simulink model "pcssp_KCURR_PFPO1_for_MUSCLE3"  (R2023b)
settings: configuration reference "configurationSettings" (kept outside this file)
undefined symbols (not defined in the file or in its folder): DiscIntNeverNeededParam, KCURR_PFPO1_fp, KCURR_PFPO1_tp, ParameterScheduling_KCURR, PCSSP_KCURR_ext_sizes
libraries: simulink x4
(part 1 of 2)
Description:
  | The KCURR_PFPO1 module implements a CS/PF current controller, including control of IpThis version performs internal gain scheduling based on an externally fed scheduling variable. Note: the coils are sorted as CS3U CS2U CS1 CS2L CS3L P1 P2 P3 P4 P5 P6
settings Model: DataDictionary=pcssp_KCURR_PFPO1.sldd  Creator=ravenst1  LastModifiedBy=grosg1
settings ConfigSetRef: SourceName=configurationSettings

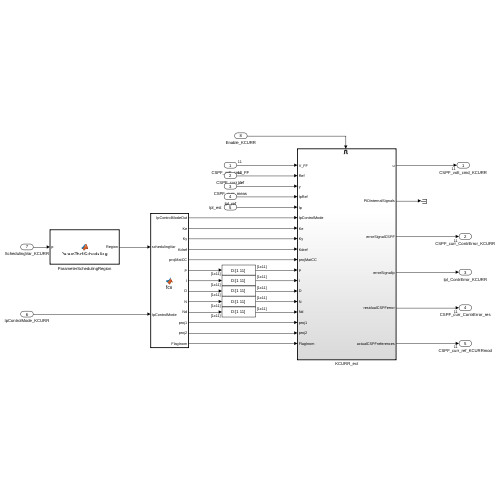
[thumbnail: Simulink's stored preview of the top-level diagram]
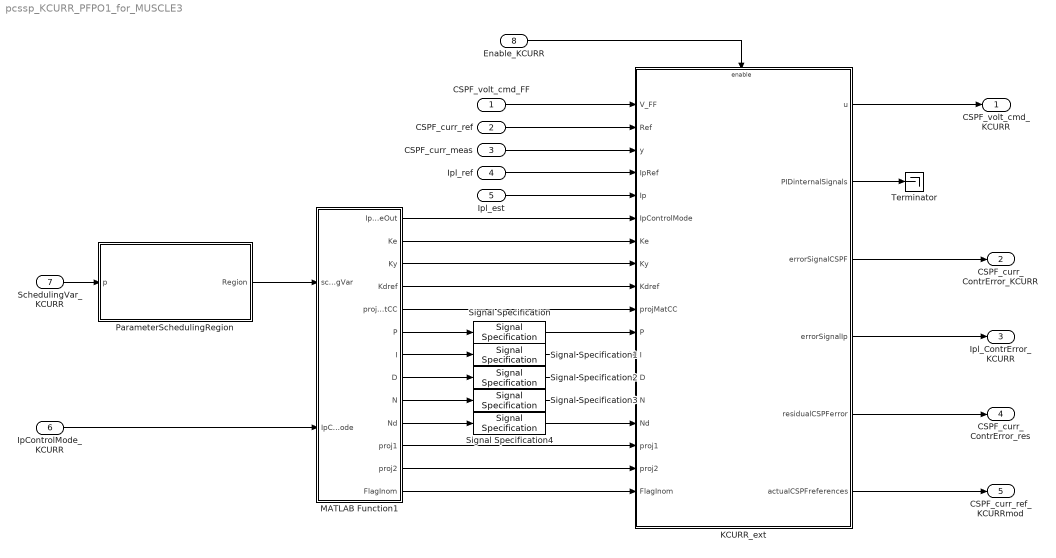
== system pcssp_KCURR_PFPO1_for_MUSCLE3 ==
  CSPF_volt_cmd_FF : Inport  PortDimensions=PCSSP_KCURR_ext_sizes.CSPF  SampleTime=KCURR_PFPO1_fp.Ts
  CSPF_curr_ref : Inport  Port=2  PortDimensions=PCSSP_KCURR_ext_sizes.CSPF  SampleTime=KCURR_PFPO1_fp.Ts
  CSPF_curr_meas : Inport  Port=3  PortDimensions=PCSSP_KCURR_ext_sizes.CSPF  SampleTime=KCURR_PFPO1_fp.Ts
  Ipl_ref : Inport  Port=4  SampleTime=KCURR_PFPO1_fp.Ts
  Ipl_est : Inport  Port=5  SampleTime=KCURR_PFPO1_fp.Ts
  IpControlMode_KCURR : Inport  Port=6  SampleTime=KCURR_PFPO1_fp.Ts
  SchedulingVar_KCURR : Inport  Port=7  PortDimensions=PCSSP_KCURR_ext_sizes.scheduling_var  SampleTime=KCURR_PFPO1_fp.Ts
  Enable_KCURR : Inport  Port=8
  KCURR_ext : Subsystem
  MATLAB Function1 : MATLAB Function  TreatAsAtomicUnit=on
  ParameterSchedulingRegion : MATLAB Function  TreatAsAtomicUnit=on
  Signal Specification{,1..4} (5 alike) : SignalSpecification  Dimensions=[1 11]
  Terminator : Terminator
  CSPF_volt_cmd_KCURR : Outport  PortDimensions=PCSSP_KCURR_ext_sizes.CSPF
  CSPF_curr_ContrError_KCURR : Outport  Port=2  PortDimensions=PCSSP_KCURR_ext_sizes.CSPF
  Ipl_ContrError_KCURR : Outport  Port=3  PortDimensions=1
  CSPF_curr_ContrError_res : Outport  Port=4  PortDimensions=PCSSP_KCURR_ext_sizes.CSPF
  CSPF_curr_ref_KCURRmod : Outport  Port=5  PortDimensions=PCSSP_KCURR_ext_sizes.CSPF
  wires:
  MATLAB Function1/10(Nd) -> Signal Specification4/1
  CSPF_curr_meas/1 -> KCURR_ext/3(y)
  MATLAB Function1/13(FlagInom) -> KCURR_ext/18(FlagInom)
  MATLAB Function1/12(proj2) -> KCURR_ext/17(proj2)
  Enable_KCURR/1 -> KCURR_ext/Enable
  MATLAB Function1/5(projMatCC) -> KCURR_ext/10(projMatCC)
  MATLAB Function1/1(IpControlModeOut) -> KCURR_ext/6(IpControlMode)
  Ipl_est/1 -> KCURR_ext/5(Ip)
  CSPF_curr_ref/1 -> KCURR_ext/2(Ref)
  ParameterSchedulingRegion/1(Region) -> MATLAB Function1/1(schedulingVar)
  CSPF_volt_cmd_FF/1 -> KCURR_ext/1(V_FF)
  MATLAB Function1/3(Ky) -> KCURR_ext/8(Ky)
  MATLAB Function1/9(N) -> Signal Specification3/1
  MATLAB Function1/4(Kdref) -> KCURR_ext/9(Kdref)
  SchedulingVar_KCURR/1 -> ParameterSchedulingRegion/1(p)
  MATLAB Function1/2(Ke) -> KCURR_ext/7(Ke)
  Ipl_ref/1 -> KCURR_ext/4(IpRef)
  IpControlMode_KCURR/1 -> MATLAB Function1/2(IpControlMode)
  MATLAB Function1/6(P) -> Signal Specification/1
  Signal Specification/1 -> KCURR_ext/11(P)
  Signal Specification1/1 -> KCURR_ext/12(I)
  MATLAB Function1/7(I) -> Signal Specification1/1
  Signal Specification2/1 -> KCURR_ext/13(D)
  MATLAB Function1/8(D) -> Signal Specification2/1
  Signal Specification3/1 -> KCURR_ext/14(N)
  Signal Specification4/1 -> KCURR_ext/15(Nd)
  MATLAB Function1/11(proj1) -> KCURR_ext/16(proj1)
  KCURR_ext/1(u) -> CSPF_volt_cmd_KCURR/1
  KCURR_ext/2(PIDinternalSignals) -> Terminator/1
  KCURR_ext/3(errorSignalCSPF) -> CSPF_curr_ContrError_KCURR/1
  KCURR_ext/4(errorSignalIp) -> Ipl_ContrError_KCURR/1
  KCURR_ext/5(residualCSPFerror) -> CSPF_curr_ContrError_res/1
  KCURR_ext/6(actualCSPFreferences) -> CSPF_curr_ref_KCURRmod/1

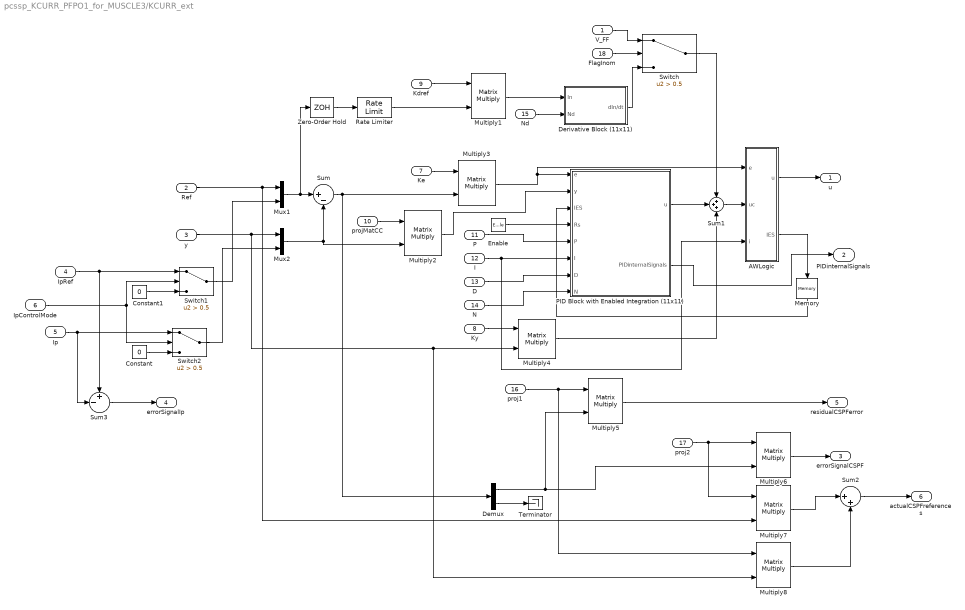
== system pcssp_KCURR_PFPO1_for_MUSCLE3/KCURR_ext ==
  V_FF : Inport
  Ref : Inport  Port=2
  y : Inport  Port=3
  IpRef : Inport  Port=4
  Ip : Inport  Port=5
  IpControlMode : Inport  Port=6
  Ke : Inport  Port=7
  Ky : Inport  Port=8
  Kdref : Inport  Port=9
  projMatCC : Inport  Port=10
  P : Inport  Port=11
  I : Inport  Port=12
  D : Inport  Port=13
  N : Inport  Port=14
  Nd : Inport  Port=15
  proj1 : Inport  Port=16
  proj2 : Inport  Port=17
  FlagInom : Inport  Port=18
  Enable : EnablePort  StatesWhenEnabling=reset  ShowOutputPort=on
  AWLogic : Subsystem
  Constant : Constant  Value=0
  Constant1 : Constant  Value=0
  Demux : Demux  Outputs=[11 1]
  Derivative Block (11x11) : Subsystem
  Memory : Memory
  Multiply{1..8} (8 alike) : Product  Inputs=**  Multiplication=Matrix(*)
  Mux1 : Mux  Inputs=2
  Mux2 : Mux  Inputs=2
  "PID Block with Enabled Integration (11x11) " : Subsystem
  Rate Limiter : RateLimiter  RisingSlewLimit=KCURR_PFPO1_tp.PosCurSlewRate  FallingSlewLimit=KCURR_PFPO1_tp.NegCurSlewRate  SampleTimeMode=inherited
  Sum : Sum  Inputs=|+-
  Sum1 : Sum  Inputs=+++
  Sum2 : Sum  Inputs=|++
  Sum3 : Sum  Inputs=+-|
  Switch : Switch  Criteria=u2 > Threshold  Threshold=0.5  SaturateOnIntegerOverflow=off  InputSameDT=off
  Switch1 : Switch  Criteria=u2 > Threshold  Threshold=0.5  SaturateOnIntegerOverflow=off  InputSameDT=off
  Switch2 : Switch  Criteria=u2 > Threshold  Threshold=0.5  SaturateOnIntegerOverflow=off  InputSameDT=off
  Terminator : Terminator
  Zero-Order Hold : ZeroOrderHold  SampleTime=KCURR_PFPO1_fp.Ts
  u : Outport
  PIDinternalSignals : Outport  Port=2
  errorSignalCSPF : Outport  Port=3
  errorSignalIp : Outport  Port=4
  residualCSPFerror : Outport  Port=5
  actualCSPFreferences : Outport  Port=6
  wires:
  N/1 -> "PID Block with Enabled Integration (11x11) "/8(N)
  D/1 -> "PID Block with Enabled Integration (11x11) "/7(D)
  I/1 -> "PID Block with Enabled Integration (11x11) "/6(I), AWLogic/3(i)
  P/1 -> "PID Block with Enabled Integration (11x11) "/5(P)
  Nd/1 -> Derivative Block (11x11)/2(Nd)
  Multiply3/1 -> AWLogic/1(e), "PID Block with Enabled Integration (11x11) "/1(e)
  "PID Block with Enabled Integration (11x11) "/2(PIDinternalSignals) -> PIDinternalSignals/1
  "PID Block with Enabled Integration (11x11) "/1(u) -> Sum1/2
  Multiply4/1 -> Sum1/3
  V_FF/1 -> Switch/1
  Switch/1 -> Sum1/1
  FlagInom/1 -> Switch/2
  Kdref/1 -> Multiply1/1
  Ke/1 -> Multiply3/1
  Ky/1 -> Multiply4/1
  Sum1/1 -> AWLogic/2(uc)
  AWLogic/1(u) -> u/1
  AWLogic/2(IES) -> Memory/1
  Enable/1 -> "PID Block with Enabled Integration (11x11) "/4(Rs)
  Memory/1 -> "PID Block with Enabled Integration (11x11) "/3(IES)
  IpRef/1 -> Sum3/1, Switch1/1
  IpControlMode/1 -> Switch2/2, Switch1/2
  Ip/1 -> Sum3/2, Switch2/1
  Constant/1 -> Switch2/3
  Constant1/1 -> Switch1/3
  Switch1/1 -> Mux1/2
  Switch2/1 -> Mux2/2
  Sum/1 -> Multiply3/2, Demux/1
  Ref/1 -> Multiply7/2, Mux1/1
  y/1 -> Multiply4/2, Multiply8/2, Mux2/1
  Mux1/1 -> Zero-Order Hold/1, Sum/1
  Mux2/1 -> Multiply2/2, Sum/2
  Multiply2/1 -> "PID Block with Enabled Integration (11x11) "/2(y)
  projMatCC/1 -> Multiply2/1
  Rate Limiter/1 -> Multiply1/2
  Multiply1/1 -> Derivative Block (11x11)/1(In)
  Derivative Block (11x11)/1(dIn/dt) -> Switch/3
  proj1/1 -> Multiply5/1, Multiply8/1
  Multiply5/1 -> residualCSPFerror/1
  proj2/1 -> Multiply7/1, Multiply6/1
  Demux/1 -> Multiply5/2, Multiply6/2
  Multiply6/1 -> errorSignalCSPF/1
  Multiply8/1 -> Sum2/2
  Multiply7/1 -> Sum2/1
  Sum2/1 -> actualCSPFreferences/1
  Sum3/1 -> errorSignalIp/1
  Demux/2 -> Terminator/1
  Zero-Order Hold/1 -> Rate Limiter/1

== system pcssp_KCURR_PFPO1_for_MUSCLE3/KCURR_ext/AWLogic ==
  e : Inport
  uc : Inport  Port=2
  i : Inport  Port=3
  Add : Sum  Inputs=+-
  Compare To Zero : simulink/Logic and Bit Operations/Compare To Zero  relop=>  OutDataTypeStr=boolean
  Compare To Zero1 : simulink/Logic and Bit Operations/Compare To Zero  relop=<  OutDataTypeStr=boolean
  Compare To Zero2 : simulink/Logic and Bit Operations/Compare To Zero  relop=>  OutDataTypeStr=boolean
  Compare To Zero3 : simulink/Logic and Bit Operations/Compare To Zero  relop=<  OutDataTypeStr=boolean
  Logical Operator : Logic  AllPortsSameDT=off  OutDataTypeStr=boolean
  Logical Operator1 : Logic  AllPortsSameDT=off  OutDataTypeStr=boolean
  Logical Operator2 : Logic  Operator=OR  AllPortsSameDT=off  OutDataTypeStr=boolean
  Logical Operator3 : Logic  Operator=NOT  Inputs=1  AllPortsSameDT=off  OutDataTypeStr=boolean
  Product : Product
  Saturation : Saturate  UpperLimit=KCURR_PFPO1_tp.Vup  LowerLimit=KCURR_PFPO1_tp.Vlow
  u : Outport
  IES : Outport  Port=2
  wires:
  Saturation/1 -> Add/2, u/1
  uc/1 -> Saturation/1, Add/1
  Add/1 -> Compare To Zero1/1, Compare To Zero/1
  e/1 -> Product/1
  Product/1 -> Compare To Zero3/1, Compare To Zero2/1
  Compare To Zero/1 -> Logical Operator/1
  Compare To Zero2/1 -> Logical Operator/2
  Compare To Zero1/1 -> Logical Operator1/1
  Compare To Zero3/1 -> Logical Operator1/2
  Logical Operator/1 -> Logical Operator2/1
  Logical Operator1/1 -> Logical Operator2/2
  Logical Operator2/1 -> Logical Operator3/1
  Logical Operator3/1 -> IES/1
  i/1 -> Product/2

== system pcssp_KCURR_PFPO1_for_MUSCLE3/KCURR_ext/Derivative Block (11x11) ==
  In : Inport  SampleTime=KCURR_PFPO1_fp.Ts
  Nd : Inport  Port=2  SampleTime=KCURR_PFPO1_fp.Ts
  Demux : Demux  Outputs=11
  Demux1 : Demux  Outputs=11
  Derivative Filter : Subsystem
  Derivative Filter1 : Subsystem
  Derivative Filter10 : Subsystem
  Derivative Filter2 : Subsystem
  Derivative Filter3 : Subsystem
  Derivative Filter4 : Subsystem
  Derivative Filter5 : Subsystem
  Derivative Filter6 : Subsystem
  Derivative Filter7 : Subsystem
  Derivative Filter8 : Subsystem
  Derivative Filter9 : Subsystem
  Mux : Mux  Inputs=11
  dIn/dt : Outport
  wires:
  Demux1/11 -> Derivative Filter10/2(nd)
  Demux1/10 -> Derivative Filter9/2(nd)
  Demux1/9 -> Derivative Filter8/2(nd)
  Demux1/8 -> Derivative Filter7/2(nd)
  Demux1/7 -> Derivative Filter6/2(nd)
  Demux1/6 -> Derivative Filter5/2(nd)
  Demux1/5 -> Derivative Filter4/2(nd)
  Demux1/4 -> Derivative Filter3/2(nd)
  Demux1/3 -> Derivative Filter2/2(nd)
  Demux1/2 -> Derivative Filter1/2(nd)
  Demux1/1 -> Derivative Filter/2(nd)
  Nd/1 -> Demux1/1
  Mux/1 -> dIn/dt/1
  Demux/6 -> Derivative Filter5/1(In)
  Derivative Filter5/1(dIn/dt) -> Mux/6
  Demux/10 -> Derivative Filter9/1(In)
  Derivative Filter10/1(dIn/dt) -> Mux/11
  Derivative Filter8/1(dIn/dt) -> Mux/9
  Derivative Filter/1(dIn/dt) -> Mux/1
  Demux/5 -> Derivative Filter4/1(In)
  Demux/9 -> Derivative Filter8/1(In)
  Demux/8 -> Derivative Filter7/1(In)
  Demux/11 -> Derivative Filter10/1(In)
  Derivative Filter3/1(dIn/dt) -> Mux/4
  Derivative Filter2/1(dIn/dt) -> Mux/3
  Derivative Filter1/1(dIn/dt) -> Mux/2
  Derivative Filter7/1(dIn/dt) -> Mux/8
  Demux/3 -> Derivative Filter2/1(In)
  Demux/4 -> Derivative Filter3/1(In)
  Demux/1 -> Derivative Filter/1(In)
  Derivative Filter4/1(dIn/dt) -> Mux/5
  Derivative Filter6/1(dIn/dt) -> Mux/7
  Derivative Filter9/1(dIn/dt) -> Mux/10
  Demux/2 -> Derivative Filter1/1(In)
  In/1 -> Demux/1
  Demux/7 -> Derivative Filter6/1(In)

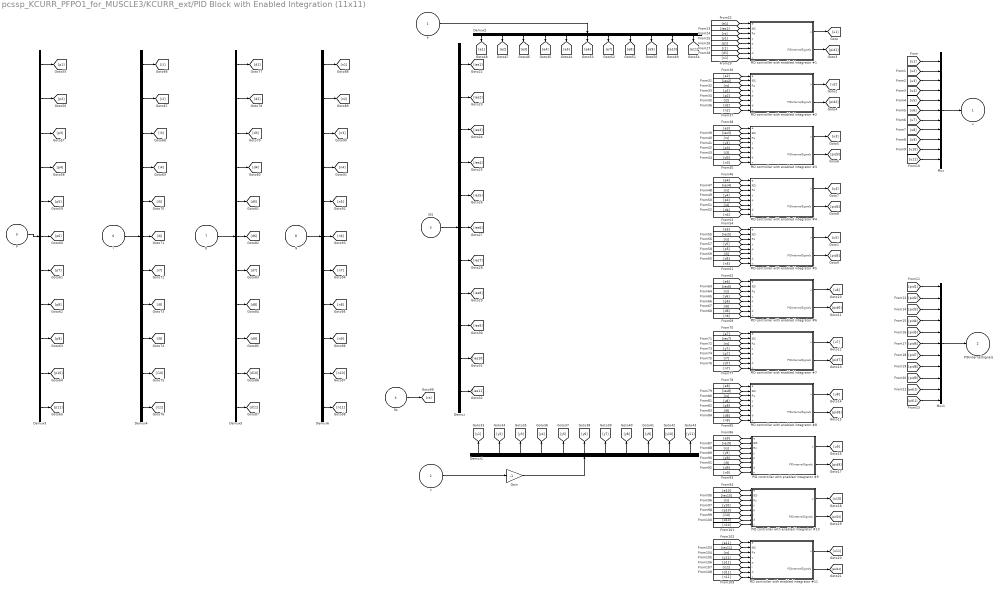
== system pcssp_KCURR_PFPO1_for_MUSCLE3/KCURR_ext/PID Block with Enabled Integration (11x11)  ==
  e : Inport
  y : Inport  Port=2
  IES : Inport  Port=3
  Rs : Inport  Port=4
  P : Inport  Port=5
  I : Inport  Port=6
  D : Inport  Port=7
  N : Inport  Port=8
  Demux{,1..6} (7 alike) : Demux  Outputs=11
  Gain : Gain  Gain=-1
  Mux : Mux  Inputs=11
  Mux1 : Mux  Inputs=11
  PID controller with enabled integrator #1 : Subsystem
  PID controller with enabled integrator #10 : Subsystem
  PID controller with enabled integrator #11 : Subsystem
  PID controller with enabled integrator #2 : Subsystem
  PID controller with enabled integrator #3 : Subsystem
  PID controller with enabled integrator #4 : Subsystem
  PID controller with enabled integrator #5 : Subsystem
  PID controller with enabled integrator #6 : Subsystem
  PID controller with enabled integrator #7 : Subsystem
  PID controller with enabled integrator #8 : Subsystem
  PID controller with enabled integrator #9 : Subsystem
  u : Outport
  PIDinternalSignals : Outport  Port=2
  wires:
  [e11] -> PID controller with enabled integrator #11/1(e)
  [rs] -> PID controller with enabled integrator #11/3(Rs)
  [ies11] -> PID controller with enabled integrator #11/2(IES)
  [p11] -> PID controller with enabled integrator #11/5(p)
  [i11] -> PID controller with enabled integrator #11/6(i)
  [n11] -> PID controller with enabled integrator #11/8(n)
  [y11] -> PID controller with enabled integrator #11/4(y)
  [d11] -> PID controller with enabled integrator #11/7(d)
  [e10] -> PID controller with enabled integrator #10/1(e)
  [rs] -> PID controller with enabled integrator #10/3(Rs)
  [ies10] -> PID controller with enabled integrator #10/2(IES)
  [p10] -> PID controller with enabled integrator #10/5(p)
  [i10] -> PID controller with enabled integrator #10/6(i)
  [n10] -> PID controller with enabled integrator #10/8(n)
  [y10] -> PID controller with enabled integrator #10/4(y)
  [d10] -> PID controller with enabled integrator #10/7(d)
  [e9] -> PID controller with enabled integrator #9/1(e)
  [rs] -> PID controller with enabled integrator #9/3(Rs)
  [ies9] -> PID controller with enabled integrator #9/2(IES)
  [p9] -> PID controller with enabled integrator #9/5(p)
  [i9] -> PID controller with enabled integrator #9/6(i)
  [n9] -> PID controller with enabled integrator #9/8(n)
  [y9] -> PID controller with enabled integrator #9/4(y)
  [d9] -> PID controller with enabled integrator #9/7(d)
  [e8] -> PID controller with enabled integrator #8/1(e)
  [rs] -> PID controller with enabled integrator #8/3(Rs)
  [ies8] -> PID controller with enabled integrator #8/2(IES)
  [p8] -> PID controller with enabled integrator #8/5(p)
  [i8] -> PID controller with enabled integrator #8/6(i)
  [n8] -> PID controller with enabled integrator #8/8(n)
  [y8] -> PID controller with enabled integrator #8/4(y)
  [d8] -> PID controller with enabled integrator #8/7(d)
  [e7] -> PID controller with enabled integrator #7/1(e)
  [rs] -> PID controller with enabled integrator #7/3(Rs)
  [ies7] -> PID controller with enabled integrator #7/2(IES)
  [p7] -> PID controller with enabled integrator #7/5(p)
  [i7] -> PID controller with enabled integrator #7/6(i)
  [n7] -> PID controller with enabled integrator #7/8(n)
  [y7] -> PID controller with enabled integrator #7/4(y)
  [d7] -> PID controller with enabled integrator #7/7(d)
  [e6] -> PID controller with enabled integrator #6/1(e)
  [rs] -> PID controller with enabled integrator #6/3(Rs)
  [ies6] -> PID controller with enabled integrator #6/2(IES)
  [p6] -> PID controller with enabled integrator #6/5(p)
  [i6] -> PID controller with enabled integrator #6/6(i)
  [n6] -> PID controller with enabled integrator #6/8(n)
  [y6] -> PID controller with enabled integrator #6/4(y)
  [d6] -> PID controller with enabled integrator #6/7(d)
  [e5] -> PID controller with enabled integrator #5/1(e)
  [rs] -> PID controller with enabled integrator #5/3(Rs)
  [ies5] -> PID controller with enabled integrator #5/2(IES)
  [p5] -> PID controller with enabled integrator #5/5(p)
  [i5] -> PID controller with enabled integrator #5/6(i)
  [n5] -> PID controller with enabled integrator #5/8(n)
  [y5] -> PID controller with enabled integrator #5/4(y)
  [d5] -> PID controller with enabled integrator #5/7(d)
  [e4] -> PID controller with enabled integrator #4/1(e)
  [rs] -> PID controller with enabled integrator #4/3(Rs)
  [ies4] -> PID controller with enabled integrator #4/2(IES)
  [p4] -> PID controller with enabled integrator #4/5(p)
  [i4] -> PID controller with enabled integrator #4/6(i)
  [n4] -> PID controller with enabled integrator #4/8(n)
  [y4] -> PID controller with enabled integrator #4/4(y)
  [d4] -> PID controller with enabled integrator #4/7(d)
  [e3] -> PID controller with enabled integrator #3/1(e)
  [rs] -> PID controller with enabled integrator #3/3(Rs)
  [ies3] -> PID controller with enabled integrator #3/2(IES)
  [p3] -> PID controller with enabled integrator #3/5(p)
  [i3] -> PID controller with enabled integrator #3/6(i)
  [n3] -> PID controller with enabled integrator #3/8(n)
  [y3] -> PID controller with enabled integrator #3/4(y)
  [d3] -> PID controller with enabled integrator #3/7(d)
  [e2] -> PID controller with enabled integrator #2/1(e)
  [rs] -> PID controller with enabled integrator #2/3(Rs)
  [ies2] -> PID controller with enabled integrator #2/2(IES)
  [p2] -> PID controller with enabled integrator #2/5(p)
  [i2] -> PID controller with enabled integrator #2/6(i)
  [n2] -> PID controller with enabled integrator #2/8(n)
  [y2] -> PID controller with enabled integrator #2/4(y)
  [d2] -> PID controller with enabled integrator #2/7(d)
  [n1] -> PID controller with enabled integrator #1/8(n)
  [d1] -> PID controller with enabled integrator #1/7(d)
  [i1] -> PID controller with enabled integrator #1/6(i)
  [p1] -> PID controller with enabled integrator #1/5(p)
  [y1] -> PID controller with enabled integrator #1/4(y)
  Rs/1 -> [rs]
  [rs] -> PID controller with enabled integrator #1/3(Rs)
  [ies1] -> PID controller with enabled integrator #1/2(IES)
  [e1] -> PID controller with enabled integrator #1/1(e)
  Demux6/1 -> [n1]
  Demux6/6 -> [n6]
  Demux6/11 -> [n11]
  Demux6/10 -> [n10]
  Demux6/7 -> [n7]
  Demux6/2 -> [n2]
  Demux6/3 -> [n3]
  Demux6/5 -> [n5]
  Demux6/9 -> [n9]
  Demux6/8 -> [n8]
  Demux6/4 -> [n4]
  N/1 -> Demux6/1
  Demux5/1 -> [d1]
  Demux5/6 -> [d6]
  Demux5/11 -> [d11]
  Demux5/10 -> [d10]
  Demux5/7 -> [d7]
  Demux5/2 -> [d2]
  Demux5/3 -> [d3]
  Demux5/5 -> [d5]
  Demux5/9 -> [d9]
  Demux5/8 -> [d8]
  Demux5/4 -> [d4]
  D/1 -> Demux5/1
  I/1 -> Demux4/1
  Demux4/1 -> [i1]
  Demux4/2 -> [i2]
  Demux4/4 -> [i4]
  Demux4/10 -> [i10]
  Demux4/6 -> [i6]
  Demux4/3 -> [i3]
  Demux4/7 -> [i7]
  Demux4/9 -> [i9]
  Demux4/8 -> [i8]
  Demux4/5 -> [i5]
  Demux4/11 -> [i11]
  Demux3/11 -> [p11]
  Demux3/10 -> [p10]
  Demux3/4 -> [p4]
  Demux3/9 -> [p9]
  Demux3/5 -> [p5]
  Demux3/1 -> [p1]
  Demux3/2 -> [p2]
  Demux3/7 -> [p7]
  Demux3/8 -> [p8]
  Demux3/3 -> [p3]
  Demux3/6 -> [p6]
  Demux2/11 -> [e11]
  Demux2/7 -> [e7]
  Demux2/9 -> [e9]
  Demux2/10 -> [e10]
  Demux2/6 -> [e6]
  Demux2/8 -> [e8]
  Demux2/5 -> [e5]
  Demux2/4 -> [e4]
  Demux2/3 -> [e3]
  Demux2/2 -> [e2]
  Demux2/1 -> [e1]
  Demux1/7 -> [y7]
  Demux1/8 -> [y8]
  Demux1/9 -> [y9]
  Demux1/10 -> [y10]
  Demux1/11 -> [y11]
  Demux1/6 -> [y6]
  Demux1/5 -> [y5]
  Demux1/4 -> [y4]
  Demux1/3 -> [y3]
  Demux1/2 -> [y2]
  Demux1/1 -> [y1]
  Demux/11 -> [ies11]
  Demux/10 -> [ies10]
  Demux/9 -> [ies9]
  Demux/8 -> [ies8]
  Demux/7 -> [ies7]
  Demux/6 -> [ies6]
  Demux/5 -> [ies5]
  Demux/4 -> [ies4]
  Demux/3 -> [ies3]
  Demux/2 -> [ies2]
  Demux/1 -> [ies1]
  [pid11] -> Mux1/11
  [pid4] -> Mux1/4
  [pid9] -> Mux1/9
  [pid7] -> Mux1/7
  [pid2] -> Mux1/2
  [pid1] -> Mux1/1
  [pid6] -> Mux1/6
  [pid3] -> Mux1/3
  [pid8] -> Mux1/8
  [pid10] -> Mux1/10
  [pid5] -> Mux1/5
  [u11] -> Mux/11
  [u10] -> Mux/10
  [u9] -> Mux/9
  [u8] -> Mux/8
  [u7] -> Mux/7
  [u6] -> Mux/6
  [u5] -> Mux/5
  [u4] -> Mux/4
  [u3] -> Mux/3
  [u2] -> Mux/2
  PID controller with enabled integrator #11/1(u) -> [u11]
  PID controller with enabled integrator #9/2(PIDinternalSignals) -> [pid9]
  PID controller with enabled integrator #11/2(PIDinternalSignals) -> [pid11]
  PID controller with enabled integrator #10/2(PIDinternalSignals) -> [pid10]
  PID controller with enabled integrator #9/1(u) -> [u9]
  PID controller with enabled integrator #10/1(u) -> [u10]
  PID controller with enabled integrator #8/1(u) -> [u8]
  PID controller with enabled integrator #8/2(PIDinternalSignals) -> [pid8]
  PID controller with enabled integrator #7/1(u) -> [u7]
  PID controller with enabled integrator #7/2(PIDinternalSignals) -> [pid7]
  PID controller with enabled integrator #6/2(PIDinternalSignals) -> [pid6]
  PID controller with enabled integrator #6/1(u) -> [u6]
  PID controller with enabled integrator #5/2(PIDinternalSignals) -> [pid5]
  PID controller with enabled integrator #4/1(u) -> [u4]
  PID controller with enabled integrator #4/2(PIDinternalSignals) -> [pid4]
  PID controller with enabled integrator #3/2(PIDinternalSignals) -> [pid3]
  PID controller with enabled integrator #3/1(u) -> [u3]
  PID controller with enabled integrator #2/2(PIDinternalSignals) -> [pid2]
  PID controller with enabled integrator #1/2(PIDinternalSignals) -> [pid1]
  PID controller with enabled integrator #2/1(u) -> [u2]
  PID controller with enabled integrator #5/1(u) -> [u5]
  PID controller with enabled integrator #1/1(u) -> [u1]
  [u1] -> Mux/1
  P/1 -> Demux3/1
  y/1 -> Gain/1
  Gain/1 -> Demux1/1
  Mux/1 -> u/1
  Mux1/1 -> PIDinternalSignals/1
  IES/1 -> Demux/1
  e/1 -> Demux2/1

== system pcssp_KCURR_PFPO1_for_MUSCLE3/KCURR_ext/Derivative Block (11x11)/Derivative Filter ==
  In : Inport
  nd : Inport  Port=2
  Filter1 : DiscreteIntegrator  DisableCoverage=on  SampleTime=-1  ICPrevOutput=DiscIntNeverNeededParam  ICPrevScaledInput=DiscIntNeverNeededParam
  Multiply3 : Product  Inputs=**
  SumD1 : Sum  DisableCoverage=on  Inputs=|+-
  dIn/dt : Outport
  wires:
  Multiply3/1 -> dIn/dt/1, Filter1/1
  nd/1 -> Multiply3/2
  In/1 -> SumD1/1
  SumD1/1 -> Multiply3/1
  Filter1/1 -> SumD1/2

== system pcssp_KCURR_PFPO1_for_MUSCLE3/KCURR_ext/Derivative Block (11x11)/Derivative Filter1 ==
  In : Inport
  nd : Inport  Port=2
  Filter1 : DiscreteIntegrator  DisableCoverage=on  SampleTime=-1  ICPrevOutput=DiscIntNeverNeededParam  ICPrevScaledInput=DiscIntNeverNeededParam
  Multiply3 : Product  Inputs=**
  SumD1 : Sum  DisableCoverage=on  Inputs=|+-
  dIn/dt : Outport
  wires:
  Multiply3/1 -> dIn/dt/1, Filter1/1
  nd/1 -> Multiply3/2
  In/1 -> SumD1/1
  SumD1/1 -> Multiply3/1
  Filter1/1 -> SumD1/2

== system pcssp_KCURR_PFPO1_for_MUSCLE3/KCURR_ext/Derivative Block (11x11)/Derivative Filter10 ==
  In : Inport
  nd : Inport  Port=2
  Filter1 : DiscreteIntegrator  DisableCoverage=on  SampleTime=-1  ICPrevOutput=DiscIntNeverNeededParam  ICPrevScaledInput=DiscIntNeverNeededParam
  Multiply3 : Product  Inputs=**
  SumD1 : Sum  DisableCoverage=on  Inputs=|+-
  dIn/dt : Outport
  wires:
  Multiply3/1 -> dIn/dt/1, Filter1/1
  nd/1 -> Multiply3/2
  In/1 -> SumD1/1
  SumD1/1 -> Multiply3/1
  Filter1/1 -> SumD1/2

== system pcssp_KCURR_PFPO1_for_MUSCLE3/KCURR_ext/Derivative Block (11x11)/Derivative Filter2 ==
  In : Inport
  nd : Inport  Port=2
  Filter1 : DiscreteIntegrator  DisableCoverage=on  SampleTime=-1  ICPrevOutput=DiscIntNeverNeededParam  ICPrevScaledInput=DiscIntNeverNeededParam
  Multiply3 : Product  Inputs=**
  SumD1 : Sum  DisableCoverage=on  Inputs=|+-
  dIn/dt : Outport
  wires:
  Multiply3/1 -> dIn/dt/1, Filter1/1
  nd/1 -> Multiply3/2
  In/1 -> SumD1/1
  SumD1/1 -> Multiply3/1
  Filter1/1 -> SumD1/2

== system pcssp_KCURR_PFPO1_for_MUSCLE3/KCURR_ext/Derivative Block (11x11)/Derivative Filter3 ==
  In : Inport
  nd : Inport  Port=2
  Filter1 : DiscreteIntegrator  DisableCoverage=on  SampleTime=-1  ICPrevOutput=DiscIntNeverNeededParam  ICPrevScaledInput=DiscIntNeverNeededParam
  Multiply3 : Product  Inputs=**
  SumD1 : Sum  DisableCoverage=on  Inputs=|+-
  dIn/dt : Outport
  wires:
  Multiply3/1 -> dIn/dt/1, Filter1/1
  nd/1 -> Multiply3/2
  In/1 -> SumD1/1
  SumD1/1 -> Multiply3/1
  Filter1/1 -> SumD1/2

== system pcssp_KCURR_PFPO1_for_MUSCLE3/KCURR_ext/Derivative Block (11x11)/Derivative Filter4 ==
  In : Inport
  nd : Inport  Port=2
  Filter1 : DiscreteIntegrator  DisableCoverage=on  SampleTime=-1  ICPrevOutput=DiscIntNeverNeededParam  ICPrevScaledInput=DiscIntNeverNeededParam
  Multiply3 : Product  Inputs=**
  SumD1 : Sum  DisableCoverage=on  Inputs=|+-
  dIn/dt : Outport
  wires:
  Multiply3/1 -> dIn/dt/1, Filter1/1
  nd/1 -> Multiply3/2
  In/1 -> SumD1/1
  SumD1/1 -> Multiply3/1
  Filter1/1 -> SumD1/2

== system pcssp_KCURR_PFPO1_for_MUSCLE3/KCURR_ext/Derivative Block (11x11)/Derivative Filter5 ==
  In : Inport
  nd : Inport  Port=2
  Filter1 : DiscreteIntegrator  DisableCoverage=on  SampleTime=-1  ICPrevOutput=DiscIntNeverNeededParam  ICPrevScaledInput=DiscIntNeverNeededParam
  Multiply3 : Product  Inputs=**
  SumD1 : Sum  DisableCoverage=on  Inputs=|+-
  dIn/dt : Outport
  wires:
  Multiply3/1 -> dIn/dt/1, Filter1/1
  nd/1 -> Multiply3/2
  In/1 -> SumD1/1
  SumD1/1 -> Multiply3/1
  Filter1/1 -> SumD1/2

== system pcssp_KCURR_PFPO1_for_MUSCLE3/KCURR_ext/Derivative Block (11x11)/Derivative Filter6 ==
  In : Inport
  nd : Inport  Port=2
  Filter1 : DiscreteIntegrator  DisableCoverage=on  SampleTime=-1  ICPrevOutput=DiscIntNeverNeededParam  ICPrevScaledInput=DiscIntNeverNeededParam
  Multiply3 : Product  Inputs=**
  SumD1 : Sum  DisableCoverage=on  Inputs=|+-
  dIn/dt : Outport
  wires:
  Multiply3/1 -> dIn/dt/1, Filter1/1
  nd/1 -> Multiply3/2
  In/1 -> SumD1/1
  SumD1/1 -> Multiply3/1
  Filter1/1 -> SumD1/2

== system pcssp_KCURR_PFPO1_for_MUSCLE3/KCURR_ext/Derivative Block (11x11)/Derivative Filter7 ==
  In : Inport
  nd : Inport  Port=2
  Filter1 : DiscreteIntegrator  DisableCoverage=on  SampleTime=-1  ICPrevOutput=DiscIntNeverNeededParam  ICPrevScaledInput=DiscIntNeverNeededParam
  Multiply3 : Product  Inputs=**
  SumD1 : Sum  DisableCoverage=on  Inputs=|+-
  dIn/dt : Outport
  wires:
  Multiply3/1 -> dIn/dt/1, Filter1/1
  nd/1 -> Multiply3/2
  In/1 -> SumD1/1
  SumD1/1 -> Multiply3/1
  Filter1/1 -> SumD1/2

== system pcssp_KCURR_PFPO1_for_MUSCLE3/KCURR_ext/Derivative Block (11x11)/Derivative Filter8 ==
  In : Inport
  nd : Inport  Port=2
  Filter1 : DiscreteIntegrator  DisableCoverage=on  SampleTime=-1  ICPrevOutput=DiscIntNeverNeededParam  ICPrevScaledInput=DiscIntNeverNeededParam
  Multiply3 : Product  Inputs=**
  SumD1 : Sum  DisableCoverage=on  Inputs=|+-
  dIn/dt : Outport
  wires:
  Multiply3/1 -> dIn/dt/1, Filter1/1
  nd/1 -> Multiply3/2
  In/1 -> SumD1/1
  SumD1/1 -> Multiply3/1
  Filter1/1 -> SumD1/2

== system pcssp_KCURR_PFPO1_for_MUSCLE3/KCURR_ext/Derivative Block (11x11)/Derivative Filter9 ==
  In : Inport
  nd : Inport  Port=2
  Filter1 : DiscreteIntegrator  DisableCoverage=on  SampleTime=-1  ICPrevOutput=DiscIntNeverNeededParam  ICPrevScaledInput=DiscIntNeverNeededParam
  Multiply3 : Product  Inputs=**
  SumD1 : Sum  DisableCoverage=on  Inputs=|+-
  dIn/dt : Outport
  wires:
  Multiply3/1 -> dIn/dt/1, Filter1/1
  nd/1 -> Multiply3/2
  In/1 -> SumD1/1
  SumD1/1 -> Multiply3/1
  Filter1/1 -> SumD1/2

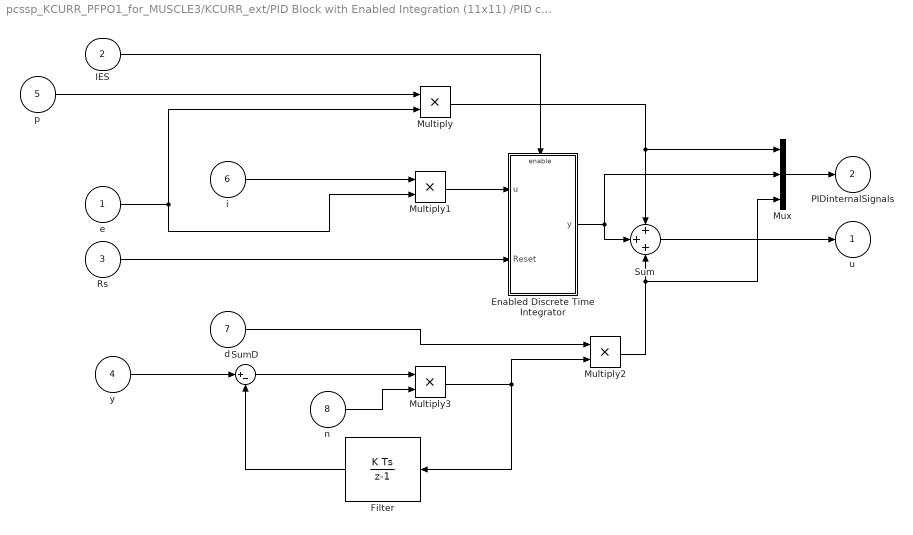
== system pcssp_KCURR_PFPO1_for_MUSCLE3/KCURR_ext/PID Block with Enabled Integration (11x11) /PID controller with enabled integrator #1 ==
  e : Inport
  IES : Inport  Port=2
  Rs : Inport  Port=3
  y : Inport  Port=4
  p : Inport  Port=5
  i : Inport  Port=6
  d : Inport  Port=7
  n : Inport  Port=8
  Enabled Discrete Time Integrator : Subsystem
  Filter : DiscreteIntegrator  DisableCoverage=on  SampleTime=-1  ICPrevOutput=DiscIntNeverNeededParam  ICPrevScaledInput=DiscIntNeverNeededParam
  Multiply{,1..3} (4 alike) : Product  Inputs=**
  Mux : Mux  Inputs=3
  Sum : Sum  Inputs=+++
  SumD : Sum  DisableCoverage=on  Inputs=|+-
  u : Outport  InitialOutput=0
  PIDinternalSignals : Outport  Port=2  InitialOutput=0
  wires:
  y/1 -> SumD/1
  i/1 -> Multiply1/1
  SumD/1 -> Multiply3/1
  n/1 -> Multiply3/2
  Multiply2/1 -> Mux/3, Sum/3
  d/1 -> Multiply2/1
  Multiply3/1 -> Filter/1, Multiply2/2
  p/1 -> Multiply/1
  Mux/1 -> PIDinternalSignals/1
  Rs/1 -> Enabled Discrete Time Integrator/2(Reset)
  e/1 -> Multiply1/2, Multiply/2
  Multiply/1 -> Mux/1, Sum/1
  Sum/1 -> u/1
  IES/1 -> Enabled Discrete Time Integrator/Enable
  Enabled Discrete Time Integrator/1(y) -> Sum/2, Mux/2
  Filter/1 -> SumD/2
  Multiply1/1 -> Enabled Discrete Time Integrator/1(u)

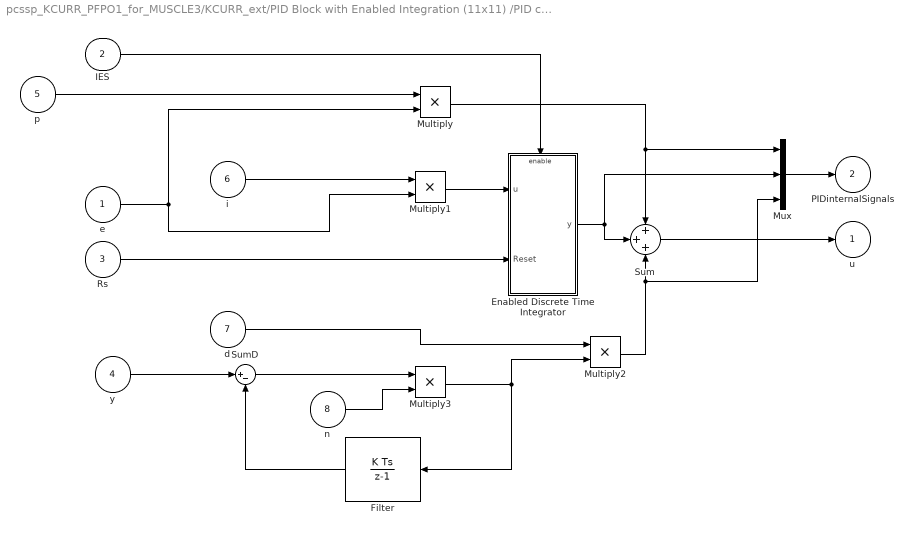
== system pcssp_KCURR_PFPO1_for_MUSCLE3/KCURR_ext/PID Block with Enabled Integration (11x11) /PID controller with enabled integrator #10 ==
  e : Inport
  IES : Inport  Port=2
  Rs : Inport  Port=3
  y : Inport  Port=4
  p : Inport  Port=5
  i : Inport  Port=6
  d : Inport  Port=7
  n : Inport  Port=8
  Enabled Discrete Time Integrator : Subsystem
  Filter : DiscreteIntegrator  DisableCoverage=on  SampleTime=-1  ICPrevOutput=DiscIntNeverNeededParam  ICPrevScaledInput=DiscIntNeverNeededParam
  Multiply{,1..3} (4 alike) : Product  Inputs=**
  Mux : Mux  Inputs=3
  Sum : Sum  Inputs=+++
  SumD : Sum  DisableCoverage=on  Inputs=|+-
  u : Outport  InitialOutput=0
  PIDinternalSignals : Outport  Port=2  InitialOutput=0
  wires:
  y/1 -> SumD/1
  i/1 -> Multiply1/1
  SumD/1 -> Multiply3/1
  n/1 -> Multiply3/2
  Multiply2/1 -> Mux/3, Sum/3
  d/1 -> Multiply2/1
  Multiply3/1 -> Filter/1, Multiply2/2
  p/1 -> Multiply/1
  Mux/1 -> PIDinternalSignals/1
  Rs/1 -> Enabled Discrete Time Integrator/2(Reset)
  e/1 -> Multiply1/2, Multiply/2
  Multiply/1 -> Mux/1, Sum/1
  Sum/1 -> u/1
  IES/1 -> Enabled Discrete Time Integrator/Enable
  Enabled Discrete Time Integrator/1(y) -> Sum/2, Mux/2
  Filter/1 -> SumD/2
  Multiply1/1 -> Enabled Discrete Time Integrator/1(u)

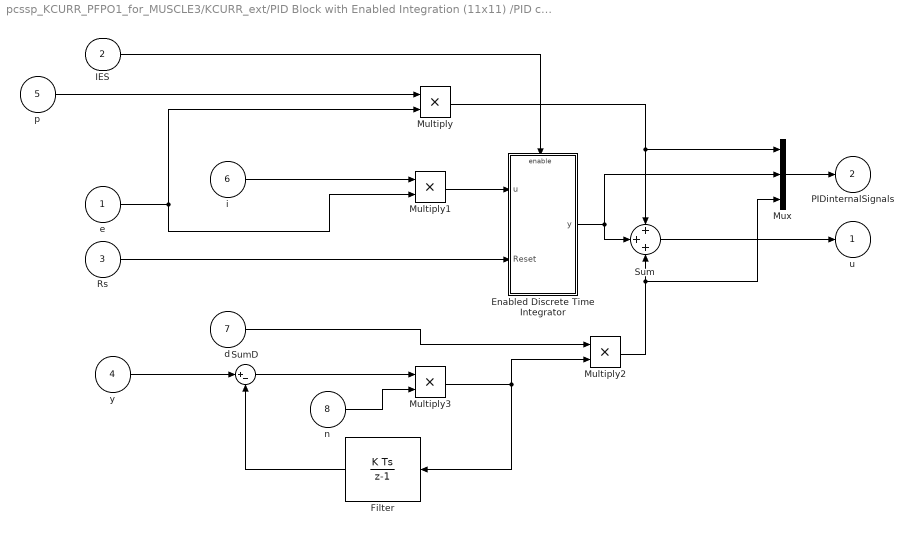
== system pcssp_KCURR_PFPO1_for_MUSCLE3/KCURR_ext/PID Block with Enabled Integration (11x11) /PID controller with enabled integrator #11 ==
  e : Inport
  IES : Inport  Port=2
  Rs : Inport  Port=3
  y : Inport  Port=4
  p : Inport  Port=5
  i : Inport  Port=6
  d : Inport  Port=7
  n : Inport  Port=8
  Enabled Discrete Time Integrator : Subsystem
  Filter : DiscreteIntegrator  DisableCoverage=on  SampleTime=-1  ICPrevOutput=DiscIntNeverNeededParam  ICPrevScaledInput=DiscIntNeverNeededParam
  Multiply{,1..3} (4 alike) : Product  Inputs=**
  Mux : Mux  Inputs=3
  Sum : Sum  Inputs=+++
  SumD : Sum  DisableCoverage=on  Inputs=|+-
  u : Outport  InitialOutput=0
  PIDinternalSignals : Outport  Port=2  InitialOutput=0
  wires:
  y/1 -> SumD/1
  i/1 -> Multiply1/1
  SumD/1 -> Multiply3/1
  n/1 -> Multiply3/2
  Multiply2/1 -> Mux/3, Sum/3
  d/1 -> Multiply2/1
  Multiply3/1 -> Filter/1, Multiply2/2
  p/1 -> Multiply/1
  Mux/1 -> PIDinternalSignals/1
  Rs/1 -> Enabled Discrete Time Integrator/2(Reset)
  e/1 -> Multiply1/2, Multiply/2
  Multiply/1 -> Mux/1, Sum/1
  Sum/1 -> u/1
  IES/1 -> Enabled Discrete Time Integrator/Enable
  Enabled Discrete Time Integrator/1(y) -> Sum/2, Mux/2
  Filter/1 -> SumD/2
  Multiply1/1 -> Enabled Discrete Time Integrator/1(u)

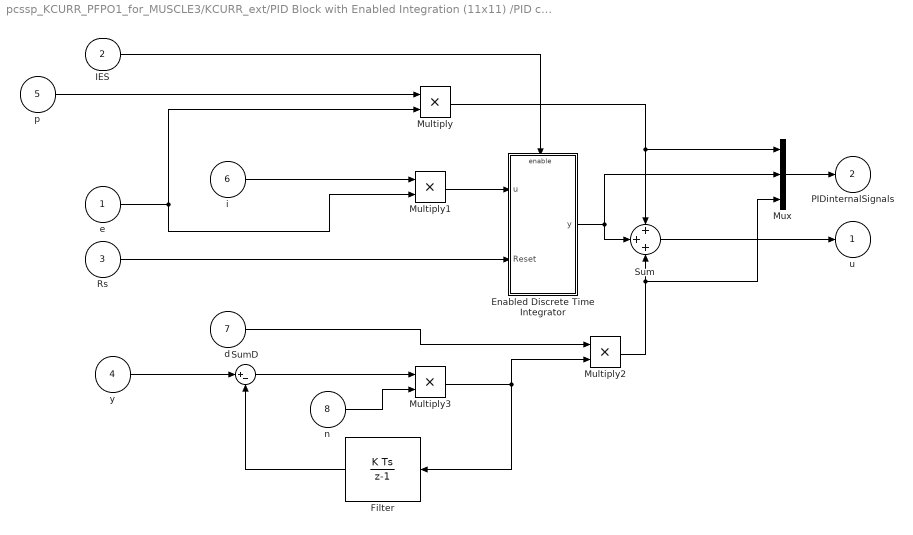
== system pcssp_KCURR_PFPO1_for_MUSCLE3/KCURR_ext/PID Block with Enabled Integration (11x11) /PID controller with enabled integrator #2 ==
  e : Inport
  IES : Inport  Port=2
  Rs : Inport  Port=3
  y : Inport  Port=4
  p : Inport  Port=5
  i : Inport  Port=6
  d : Inport  Port=7
  n : Inport  Port=8
  Enabled Discrete Time Integrator : Subsystem
  Filter : DiscreteIntegrator  DisableCoverage=on  SampleTime=-1  ICPrevOutput=DiscIntNeverNeededParam  ICPrevScaledInput=DiscIntNeverNeededParam
  Multiply{,1..3} (4 alike) : Product  Inputs=**
  Mux : Mux  Inputs=3
  Sum : Sum  Inputs=+++
  SumD : Sum  DisableCoverage=on  Inputs=|+-
  u : Outport  InitialOutput=0
  PIDinternalSignals : Outport  Port=2  InitialOutput=0
  wires:
  y/1 -> SumD/1
  i/1 -> Multiply1/1
  SumD/1 -> Multiply3/1
  n/1 -> Multiply3/2
  Multiply2/1 -> Mux/3, Sum/3
  d/1 -> Multiply2/1
  Multiply3/1 -> Filter/1, Multiply2/2
  p/1 -> Multiply/1
  Mux/1 -> PIDinternalSignals/1
  Rs/1 -> Enabled Discrete Time Integrator/2(Reset)
  e/1 -> Multiply1/2, Multiply/2
  Multiply/1 -> Mux/1, Sum/1
  Sum/1 -> u/1
  IES/1 -> Enabled Discrete Time Integrator/Enable
  Enabled Discrete Time Integrator/1(y) -> Sum/2, Mux/2
  Filter/1 -> SumD/2
  Multiply1/1 -> Enabled Discrete Time Integrator/1(u)

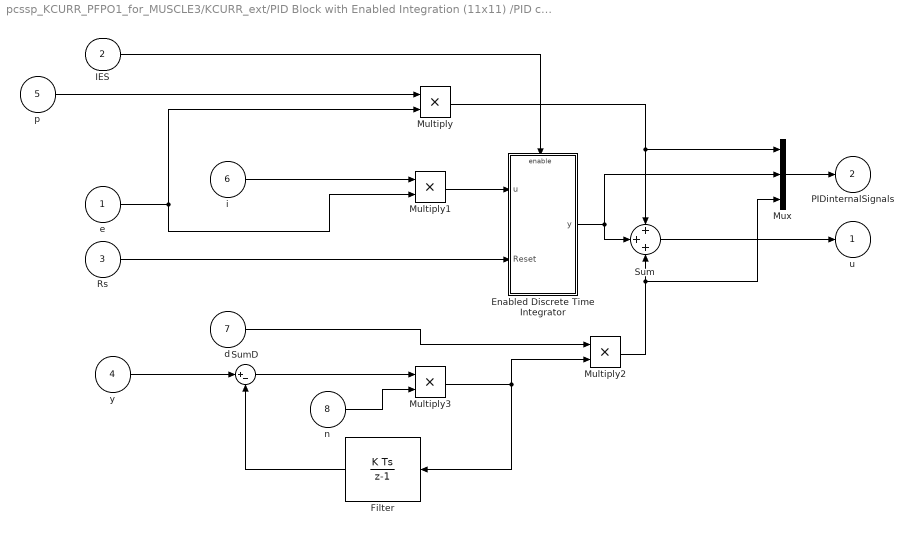
== system pcssp_KCURR_PFPO1_for_MUSCLE3/KCURR_ext/PID Block with Enabled Integration (11x11) /PID controller with enabled integrator #3 ==
  e : Inport
  IES : Inport  Port=2
  Rs : Inport  Port=3
  y : Inport  Port=4
  p : Inport  Port=5
  i : Inport  Port=6
  d : Inport  Port=7
  n : Inport  Port=8
  Enabled Discrete Time Integrator : Subsystem
  Filter : DiscreteIntegrator  DisableCoverage=on  SampleTime=-1  ICPrevOutput=DiscIntNeverNeededParam  ICPrevScaledInput=DiscIntNeverNeededParam
  Multiply{,1..3} (4 alike) : Product  Inputs=**
  Mux : Mux  Inputs=3
  Sum : Sum  Inputs=+++
  SumD : Sum  DisableCoverage=on  Inputs=|+-
  u : Outport  InitialOutput=0
  PIDinternalSignals : Outport  Port=2  InitialOutput=0
  wires:
  y/1 -> SumD/1
  i/1 -> Multiply1/1
  SumD/1 -> Multiply3/1
  n/1 -> Multiply3/2
  Multiply2/1 -> Mux/3, Sum/3
  d/1 -> Multiply2/1
  Multiply3/1 -> Filter/1, Multiply2/2
  p/1 -> Multiply/1
  Mux/1 -> PIDinternalSignals/1
  Rs/1 -> Enabled Discrete Time Integrator/2(Reset)
  e/1 -> Multiply1/2, Multiply/2
  Multiply/1 -> Mux/1, Sum/1
  Sum/1 -> u/1
  IES/1 -> Enabled Discrete Time Integrator/Enable
  Enabled Discrete Time Integrator/1(y) -> Sum/2, Mux/2
  Filter/1 -> SumD/2
  Multiply1/1 -> Enabled Discrete Time Integrator/1(u)

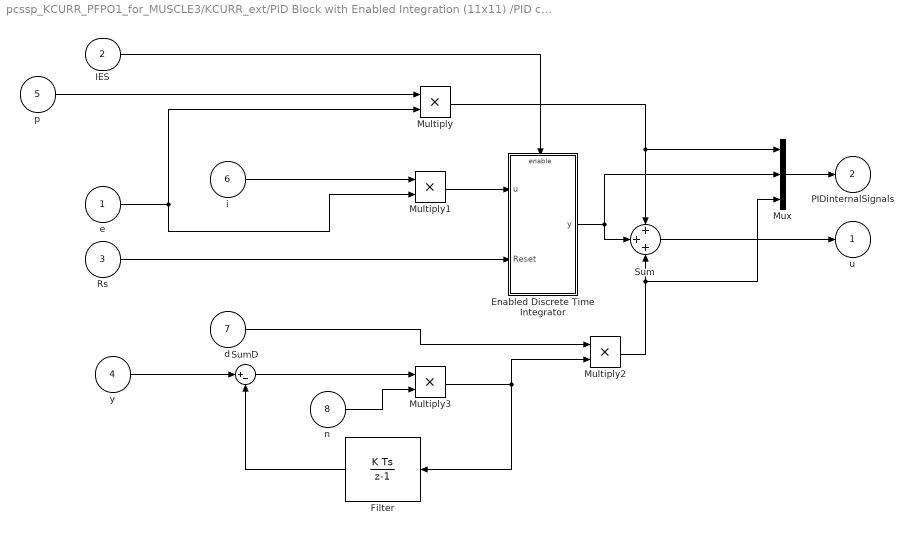
== system pcssp_KCURR_PFPO1_for_MUSCLE3/KCURR_ext/PID Block with Enabled Integration (11x11) /PID controller with enabled integrator #4 ==
  e : Inport
  IES : Inport  Port=2
  Rs : Inport  Port=3
  y : Inport  Port=4
  p : Inport  Port=5
  i : Inport  Port=6
  d : Inport  Port=7
  n : Inport  Port=8
  Enabled Discrete Time Integrator : Subsystem
  Filter : DiscreteIntegrator  DisableCoverage=on  SampleTime=-1  ICPrevOutput=DiscIntNeverNeededParam  ICPrevScaledInput=DiscIntNeverNeededParam
  Multiply{,1..3} (4 alike) : Product  Inputs=**
  Mux : Mux  Inputs=3
  Sum : Sum  Inputs=+++
  SumD : Sum  DisableCoverage=on  Inputs=|+-
  u : Outport  InitialOutput=0
  PIDinternalSignals : Outport  Port=2  InitialOutput=0
  wires:
  y/1 -> SumD/1
  i/1 -> Multiply1/1
  SumD/1 -> Multiply3/1
  n/1 -> Multiply3/2
  Multiply2/1 -> Mux/3, Sum/3
  d/1 -> Multiply2/1
  Multiply3/1 -> Filter/1, Multiply2/2
  p/1 -> Multiply/1
  Mux/1 -> PIDinternalSignals/1
  Rs/1 -> Enabled Discrete Time Integrator/2(Reset)
  e/1 -> Multiply1/2, Multiply/2
  Multiply/1 -> Mux/1, Sum/1
  Sum/1 -> u/1
  IES/1 -> Enabled Discrete Time Integrator/Enable
  Enabled Discrete Time Integrator/1(y) -> Sum/2, Mux/2
  Filter/1 -> SumD/2
  Multiply1/1 -> Enabled Discrete Time Integrator/1(u)

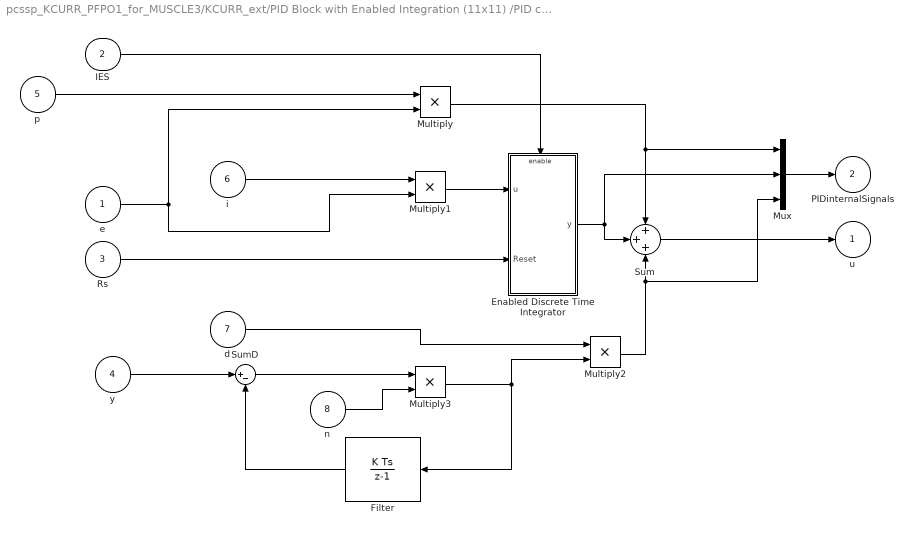
== system pcssp_KCURR_PFPO1_for_MUSCLE3/KCURR_ext/PID Block with Enabled Integration (11x11) /PID controller with enabled integrator #5 ==
  e : Inport
  IES : Inport  Port=2
  Rs : Inport  Port=3
  y : Inport  Port=4
  p : Inport  Port=5
  i : Inport  Port=6
  d : Inport  Port=7
  n : Inport  Port=8
  Enabled Discrete Time Integrator : Subsystem
  Filter : DiscreteIntegrator  DisableCoverage=on  SampleTime=-1  ICPrevOutput=DiscIntNeverNeededParam  ICPrevScaledInput=DiscIntNeverNeededParam
  Multiply{,1..3} (4 alike) : Product  Inputs=**
  Mux : Mux  Inputs=3
  Sum : Sum  Inputs=+++
  SumD : Sum  DisableCoverage=on  Inputs=|+-
  u : Outport  InitialOutput=0
  PIDinternalSignals : Outport  Port=2  InitialOutput=0
  wires:
  y/1 -> SumD/1
  i/1 -> Multiply1/1
  SumD/1 -> Multiply3/1
  n/1 -> Multiply3/2
  Multiply2/1 -> Mux/3, Sum/3
  d/1 -> Multiply2/1
  Multiply3/1 -> Filter/1, Multiply2/2
  p/1 -> Multiply/1
  Mux/1 -> PIDinternalSignals/1
  Rs/1 -> Enabled Discrete Time Integrator/2(Reset)
  e/1 -> Multiply1/2, Multiply/2
  Multiply/1 -> Mux/1, Sum/1
  Sum/1 -> u/1
  IES/1 -> Enabled Discrete Time Integrator/Enable
  Enabled Discrete Time Integrator/1(y) -> Sum/2, Mux/2
  Filter/1 -> SumD/2
  Multiply1/1 -> Enabled Discrete Time Integrator/1(u)

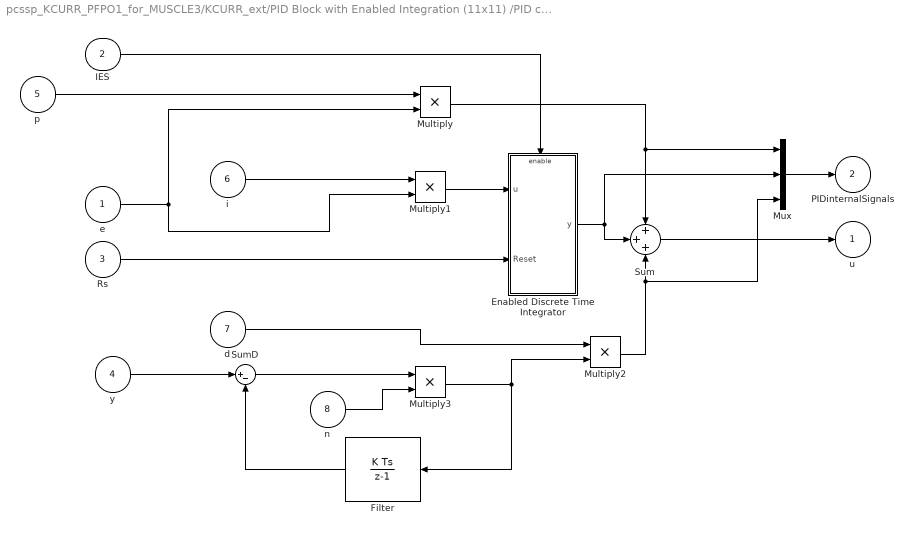
== system pcssp_KCURR_PFPO1_for_MUSCLE3/KCURR_ext/PID Block with Enabled Integration (11x11) /PID controller with enabled integrator #6 ==
  e : Inport
  IES : Inport  Port=2
  Rs : Inport  Port=3
  y : Inport  Port=4
  p : Inport  Port=5
  i : Inport  Port=6
  d : Inport  Port=7
  n : Inport  Port=8
  Enabled Discrete Time Integrator : Subsystem
  Filter : DiscreteIntegrator  DisableCoverage=on  SampleTime=-1  ICPrevOutput=DiscIntNeverNeededParam  ICPrevScaledInput=DiscIntNeverNeededParam
  Multiply{,1..3} (4 alike) : Product  Inputs=**
  Mux : Mux  Inputs=3
  Sum : Sum  Inputs=+++
  SumD : Sum  DisableCoverage=on  Inputs=|+-
  u : Outport  InitialOutput=0
  PIDinternalSignals : Outport  Port=2  InitialOutput=0
  wires:
  y/1 -> SumD/1
  i/1 -> Multiply1/1
  SumD/1 -> Multiply3/1
  n/1 -> Multiply3/2
  Multiply2/1 -> Mux/3, Sum/3
  d/1 -> Multiply2/1
  Multiply3/1 -> Filter/1, Multiply2/2
  p/1 -> Multiply/1
  Mux/1 -> PIDinternalSignals/1
  Rs/1 -> Enabled Discrete Time Integrator/2(Reset)
  e/1 -> Multiply1/2, Multiply/2
  Multiply/1 -> Mux/1, Sum/1
  Sum/1 -> u/1
  IES/1 -> Enabled Discrete Time Integrator/Enable
  Enabled Discrete Time Integrator/1(y) -> Sum/2, Mux/2
  Filter/1 -> SumD/2
  Multiply1/1 -> Enabled Discrete Time Integrator/1(u)

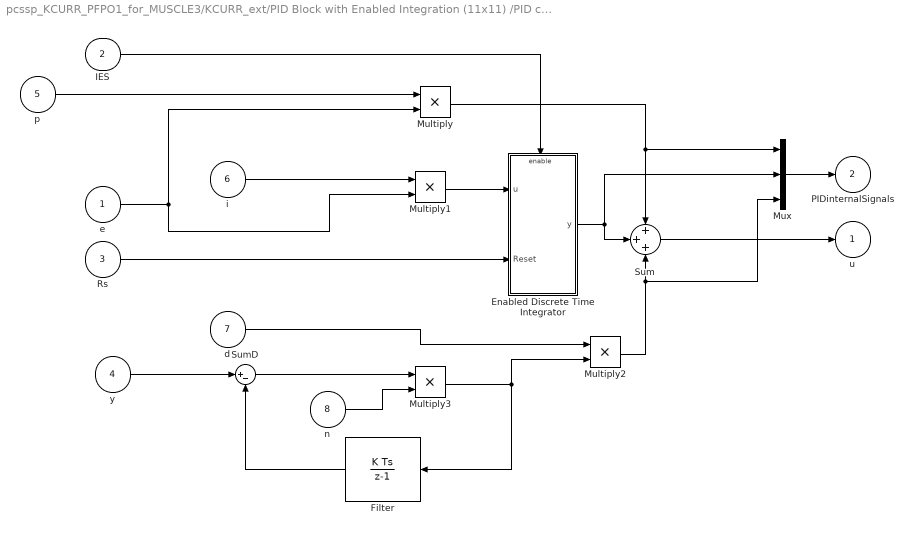
== system pcssp_KCURR_PFPO1_for_MUSCLE3/KCURR_ext/PID Block with Enabled Integration (11x11) /PID controller with enabled integrator #7 ==
  e : Inport
  IES : Inport  Port=2
  Rs : Inport  Port=3
  y : Inport  Port=4
  p : Inport  Port=5
  i : Inport  Port=6
  d : Inport  Port=7
  n : Inport  Port=8
  Enabled Discrete Time Integrator : Subsystem
  Filter : DiscreteIntegrator  DisableCoverage=on  SampleTime=-1  ICPrevOutput=DiscIntNeverNeededParam  ICPrevScaledInput=DiscIntNeverNeededParam
  Multiply{,1..3} (4 alike) : Product  Inputs=**
  Mux : Mux  Inputs=3
  Sum : Sum  Inputs=+++
  SumD : Sum  DisableCoverage=on  Inputs=|+-
  u : Outport  InitialOutput=0
  PIDinternalSignals : Outport  Port=2  InitialOutput=0
  wires:
  y/1 -> SumD/1
  i/1 -> Multiply1/1
  SumD/1 -> Multiply3/1
  n/1 -> Multiply3/2
  Multiply2/1 -> Mux/3, Sum/3
  d/1 -> Multiply2/1
  Multiply3/1 -> Filter/1, Multiply2/2
  p/1 -> Multiply/1
  Mux/1 -> PIDinternalSignals/1
  Rs/1 -> Enabled Discrete Time Integrator/2(Reset)
  e/1 -> Multiply1/2, Multiply/2
  Multiply/1 -> Mux/1, Sum/1
  Sum/1 -> u/1
  IES/1 -> Enabled Discrete Time Integrator/Enable
  Enabled Discrete Time Integrator/1(y) -> Sum/2, Mux/2
  Filter/1 -> SumD/2
  Multiply1/1 -> Enabled Discrete Time Integrator/1(u)

== system pcssp_KCURR_PFPO1_for_MUSCLE3/KCURR_ext/PID Block with Enabled Integration (11x11) /PID controller with enabled integrator #8 ==
  e : Inport
  IES : Inport  Port=2
  Rs : Inport  Port=3
  y : Inport  Port=4
  p : Inport  Port=5
  i : Inport  Port=6
  d : Inport  Port=7
  n : Inport  Port=8
  Enabled Discrete Time Integrator : Subsystem
  Filter : DiscreteIntegrator  DisableCoverage=on  SampleTime=-1  ICPrevOutput=DiscIntNeverNeededParam  ICPrevScaledInput=DiscIntNeverNeededParam
  Multiply{,1..3} (4 alike) : Product  Inputs=**
  Mux : Mux  Inputs=3
  Sum : Sum  Inputs=+++
  SumD : Sum  DisableCoverage=on  Inputs=|+-
  u : Outport  InitialOutput=0
  PIDinternalSignals : Outport  Port=2  InitialOutput=0
  wires:
  y/1 -> SumD/1
  i/1 -> Multiply1/1
  SumD/1 -> Multiply3/1
  n/1 -> Multiply3/2
  Multiply2/1 -> Mux/3, Sum/3
  d/1 -> Multiply2/1
  Multiply3/1 -> Filter/1, Multiply2/2
  p/1 -> Multiply/1
  Mux/1 -> PIDinternalSignals/1
  Rs/1 -> Enabled Discrete Time Integrator/2(Reset)
  e/1 -> Multiply1/2, Multiply/2
  Multiply/1 -> Mux/1, Sum/1
  Sum/1 -> u/1
  IES/1 -> Enabled Discrete Time Integrator/Enable
  Enabled Discrete Time Integrator/1(y) -> Sum/2, Mux/2
  Filter/1 -> SumD/2
  Multiply1/1 -> Enabled Discrete Time Integrator/1(u)

== system pcssp_KCURR_PFPO1_for_MUSCLE3/KCURR_ext/PID Block with Enabled Integration (11x11) /PID controller with enabled integrator #9 ==
  e : Inport
  IES : Inport  Port=2
  Rs : Inport  Port=3
  y : Inport  Port=4
  p : Inport  Port=5
  i : Inport  Port=6
  d : Inport  Port=7
  n : Inport  Port=8
  Enabled Discrete Time Integrator : Subsystem
  Filter : DiscreteIntegrator  DisableCoverage=on  SampleTime=-1  ICPrevOutput=DiscIntNeverNeededParam  ICPrevScaledInput=DiscIntNeverNeededParam
  Multiply{,1..3} (4 alike) : Product  Inputs=**
  Mux : Mux  Inputs=3
  Sum : Sum  Inputs=+++
  SumD : Sum  DisableCoverage=on  Inputs=|+-
  u : Outport  InitialOutput=0
  PIDinternalSignals : Outport  Port=2  InitialOutput=0
  wires:
  y/1 -> SumD/1
  i/1 -> Multiply1/1
  SumD/1 -> Multiply3/1
  n/1 -> Multiply3/2
  Multiply2/1 -> Mux/3, Sum/3
  d/1 -> Multiply2/1
  Multiply3/1 -> Filter/1, Multiply2/2
  p/1 -> Multiply/1
  Mux/1 -> PIDinternalSignals/1
  Rs/1 -> Enabled Discrete Time Integrator/2(Reset)
  e/1 -> Multiply1/2, Multiply/2
  Multiply/1 -> Mux/1, Sum/1
  Sum/1 -> u/1
  IES/1 -> Enabled Discrete Time Integrator/Enable
  Enabled Discrete Time Integrator/1(y) -> Sum/2, Mux/2
  Filter/1 -> SumD/2
  Multiply1/1 -> Enabled Discrete Time Integrator/1(u)

== system pcssp_KCURR_PFPO1_for_MUSCLE3/KCURR_ext/PID Block with Enabled Integration (11x11) /PID controller with enabled integrator #1/Enabled Discrete Time Integrator ==
  u : Inport
  Reset : Inport  Port=2
  Enable : EnablePort
  Filter : DiscreteIntegrator  DisableCoverage=on  ExternalReset=rising  SampleTime=-1  ICPrevOutput=DiscIntNeverNeededParam  ICPrevScaledInput=DiscIntNeverNeededParam
  y : Outport
  wires:
  u/1 -> Filter/1
  Filter/1 -> y/1
  Reset/1 -> Filter/2

== system pcssp_KCURR_PFPO1_for_MUSCLE3/KCURR_ext/PID Block with Enabled Integration (11x11) /PID controller with enabled integrator #10/Enabled Discrete Time Integrator ==
  u : Inport
  Reset : Inport  Port=2
  Enable : EnablePort
  Filter : DiscreteIntegrator  DisableCoverage=on  ExternalReset=rising  SampleTime=-1  ICPrevOutput=DiscIntNeverNeededParam  ICPrevScaledInput=DiscIntNeverNeededParam
  y : Outport
  wires:
  u/1 -> Filter/1
  Filter/1 -> y/1
  Reset/1 -> Filter/2

== system pcssp_KCURR_PFPO1_for_MUSCLE3/KCURR_ext/PID Block with Enabled Integration (11x11) /PID controller with enabled integrator #11/Enabled Discrete Time Integrator ==
  u : Inport
  Reset : Inport  Port=2
  Enable : EnablePort
  Filter : DiscreteIntegrator  DisableCoverage=on  ExternalReset=rising  SampleTime=-1  ICPrevOutput=DiscIntNeverNeededParam  ICPrevScaledInput=DiscIntNeverNeededParam
  y : Outport
  wires:
  u/1 -> Filter/1
  Filter/1 -> y/1
  Reset/1 -> Filter/2

== system pcssp_KCURR_PFPO1_for_MUSCLE3/KCURR_ext/PID Block with Enabled Integration (11x11) /PID controller with enabled integrator #2/Enabled Discrete Time Integrator ==
  u : Inport
  Reset : Inport  Port=2
  Enable : EnablePort
  Filter : DiscreteIntegrator  DisableCoverage=on  ExternalReset=rising  SampleTime=-1  ICPrevOutput=DiscIntNeverNeededParam  ICPrevScaledInput=DiscIntNeverNeededParam
  y : Outport
  wires:
  u/1 -> Filter/1
  Filter/1 -> y/1
  Reset/1 -> Filter/2

== system pcssp_KCURR_PFPO1_for_MUSCLE3/KCURR_ext/PID Block with Enabled Integration (11x11) /PID controller with enabled integrator #3/Enabled Discrete Time Integrator ==
  u : Inport
  Reset : Inport  Port=2
  Enable : EnablePort
  Filter : DiscreteIntegrator  DisableCoverage=on  ExternalReset=rising  SampleTime=-1  ICPrevOutput=DiscIntNeverNeededParam  ICPrevScaledInput=DiscIntNeverNeededParam
  y : Outport
  wires:
  u/1 -> Filter/1
  Filter/1 -> y/1
  Reset/1 -> Filter/2

== system pcssp_KCURR_PFPO1_for_MUSCLE3/KCURR_ext/PID Block with Enabled Integration (11x11) /PID controller with enabled integrator #4/Enabled Discrete Time Integrator ==
  u : Inport
  Reset : Inport  Port=2
  Enable : EnablePort
  Filter : DiscreteIntegrator  DisableCoverage=on  ExternalReset=rising  SampleTime=-1  ICPrevOutput=DiscIntNeverNeededParam  ICPrevScaledInput=DiscIntNeverNeededParam
  y : Outport
  wires:
  u/1 -> Filter/1
  Filter/1 -> y/1
  Reset/1 -> Filter/2

== system pcssp_KCURR_PFPO1_for_MUSCLE3/KCURR_ext/PID Block with Enabled Integration (11x11) /PID controller with enabled integrator #5/Enabled Discrete Time Integrator ==
  u : Inport
  Reset : Inport  Port=2
  Enable : EnablePort
  Filter : DiscreteIntegrator  DisableCoverage=on  ExternalReset=rising  SampleTime=-1  ICPrevOutput=DiscIntNeverNeededParam  ICPrevScaledInput=DiscIntNeverNeededParam
  y : Outport
  wires:
  u/1 -> Filter/1
  Filter/1 -> y/1
  Reset/1 -> Filter/2

== system pcssp_KCURR_PFPO1_for_MUSCLE3/KCURR_ext/PID Block with Enabled Integration (11x11) /PID controller with enabled integrator #6/Enabled Discrete Time Integrator ==
  u : Inport
  Reset : Inport  Port=2
  Enable : EnablePort
  Filter : DiscreteIntegrator  DisableCoverage=on  ExternalReset=rising  SampleTime=-1  ICPrevOutput=DiscIntNeverNeededParam  ICPrevScaledInput=DiscIntNeverNeededParam
  y : Outport
  wires:
  u/1 -> Filter/1
  Filter/1 -> y/1
  Reset/1 -> Filter/2

== system pcssp_KCURR_PFPO1_for_MUSCLE3/KCURR_ext/PID Block with Enabled Integration (11x11) /PID controller with enabled integrator #7/Enabled Discrete Time Integrator ==
  u : Inport
  Reset : Inport  Port=2
  Enable : EnablePort
  Filter : DiscreteIntegrator  DisableCoverage=on  ExternalReset=rising  SampleTime=-1  ICPrevOutput=DiscIntNeverNeededParam  ICPrevScaledInput=DiscIntNeverNeededParam
  y : Outport
  wires:
  u/1 -> Filter/1
  Filter/1 -> y/1
  Reset/1 -> Filter/2

== system pcssp_KCURR_PFPO1_for_MUSCLE3/KCURR_ext/PID Block with Enabled Integration (11x11) /PID controller with enabled integrator #8/Enabled Discrete Time Integrator ==
  u : Inport
  Reset : Inport  Port=2
  Enable : EnablePort
  Filter : DiscreteIntegrator  DisableCoverage=on  ExternalReset=rising  SampleTime=-1  ICPrevOutput=DiscIntNeverNeededParam  ICPrevScaledInput=DiscIntNeverNeededParam
  y : Outport
  wires:
  u/1 -> Filter/1
  Filter/1 -> y/1
  Reset/1 -> Filter/2

== system pcssp_KCURR_PFPO1_for_MUSCLE3/KCURR_ext/PID Block with Enabled Integration (11x11) /PID controller with enabled integrator #9/Enabled Discrete Time Integrator ==
  u : Inport
  Reset : Inport  Port=2
  Enable : EnablePort
  Filter : DiscreteIntegrator  DisableCoverage=on  ExternalReset=rising  SampleTime=-1  ICPrevOutput=DiscIntNeverNeededParam  ICPrevScaledInput=DiscIntNeverNeededParam
  y : Outport
  wires:
  u/1 -> Filter/1
  Filter/1 -> y/1
  Reset/1 -> Filter/2

== matlab function pcssp_KCURR_PFPO1_for_MUSCLE3/MATLAB Function1 ==
  data: schedulingVar input; IpControlModeOut output; IpControlMode input; Ke output; Ky output; Kdref output; projMatCC output; P output; I output; D output; N output; Nd output; proj1 output; proj2 output; FlagInom output; KCURR_PFPO1_Gains parameter
function [IpControlModeOut,Ke,Ky,Kdref,projMatCC,P,I,D,N,Nd,proj1,proj2,FlagInom] = fcn(schedulingVar,IpControlMode,KCURR_PFPO1_Gains)

IpControlModeOut=IpControlMode;


if IpControlMode<0.5
    Ke = KCURR_PFPO1_Gains(schedulingVar).Ke_noIp;
    Ky = KCURR_PFPO1_Gains(schedulingVar).Ky_noIp;
    Kdref = KCURR_PFPO1_Gains(schedulingVar).Kdref_noIp;
    projMatCC=KCURR_PFPO1_Gains(schedulingVar).projMatCC_noIp;
    P = KCURR_PFPO1_Gains(schedulingVar).P_noIp;
    I = KCURR_PFPO1_Gains(schedulingVar).I_noIp;
    D = KCURR_PFPO1_Gains(schedulingVar).D_noIp;
    N = KCURR_PFPO1_Gains(schedulingVar).N_noIp;
    Nd = KCURR_PFPO1_Gains(schedulingVar).Nd_noIp;
    FlagInom = KCURR_PFPO1_Gains(schedulingVar).FlagInom_noIp;
    proj1=KCURR_PFPO1_Gains(schedulingVar).proj1_noIp;
    proj2=KCURR_PFPO1_Gains(schedulingVar).proj2_noIp;
else
    Ke = KCURR_PFPO1_Gains(schedulingVar).Ke_Ip;
    Ky = KCURR_PFPO1_Gains(schedulingVar).Ky_Ip;
    Kdref = KCURR_PFPO1_Gains(schedulingVar).Kdref_Ip;
    projMatCC=KCURR_PFPO1_Gains(schedulingVar).projMatCC_Ip;
    P = KCURR_PFPO1_Gains(schedulingVar).P_Ip;
    I = KCURR_PFPO1_Gains(schedulingVar).I_Ip;
    D = KCURR_PFPO1_Gains(schedulingVar).D_Ip;
    N = KCURR_PFPO1_Gains(schedulingVar).N_Ip;
    Nd = KCURR_PFPO1_Gains(schedulingVar).Nd_Ip;
    FlagInom = KCURR_PFPO1_Gains(schedulingVar).FlagInom_Ip;
    proj1=KCURR_PFPO1_Gains(schedulingVar).proj1_Ip;
    proj2=KCURR_PFPO1_Gains(schedulingVar).proj2_Ip;
end
